simulink library "VehicleMdl"  (R2018b)
settings: Solver=VariableStepAuto  StartTime=0.0  StopTime=10.0  RelTol=1e-3
settings Model: Creator=Haraszti Sándor  LastModifiedBy=Haraszti Sándor

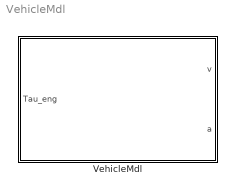
== system VehicleMdl ==
  VehicleMdl : Subsystem  mask{v_max=25, v_min=0, a_max=3, a_min=-3}
      mask prompts: v_max "v_max [m/s]"; v_min "v_min [m/s]"; a_max "a_max [m/s^2]"; a_min "a_min [m/s^2]"

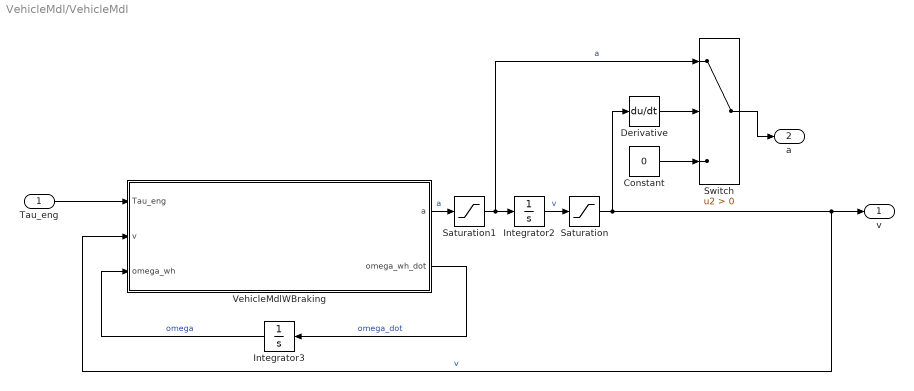
== system VehicleMdl/VehicleMdl ==
  Tau_eng : Inport
  Constant : Constant  Value=0
  Derivative : Derivative
  Integrator2 : Integrator
  Integrator3 : Integrator
  Saturation : Saturate  UpperLimit=v_max  LowerLimit=v_min
  Saturation1 : Saturate  UpperLimit=a_max  LowerLimit=a_min
  Switch : Switch  Criteria=u2 > Threshold
  VehicleMdlWBraking : MATLAB Function  TreatAsAtomicUnit=on
  v : Outport
  a : Outport  Port=2
  wires:
  Constant/1 -> Switch/3
  Switch/1 -> a/1
  Derivative/1 -> Switch/2
  Saturation1/1 -> Integrator2/1, Switch/1  "a"
  VehicleMdlWBraking/1(a) -> Saturation1/1  "a"
  VehicleMdlWBraking/2(omega_wh_dot) -> Integrator3/1  "omega_dot"
  Integrator3/1 -> VehicleMdlWBraking/3(omega_wh)  "omega"
  Saturation/1 -> Derivative/1, v/1, VehicleMdlWBraking/2(v)  "v"
  Tau_eng/1 -> VehicleMdlWBraking/1(Tau_eng)
  Integrator2/1 -> Saturation/1  "v"

== matlab function VehicleMdl/VehicleMdlWBraking ==
  data: Tau_eng input; a output; v input; omega_wh input; omega_wh_dot output
function [a, omega_wh_dot] = vehicleMdl(Tau_eng, v, omega_wh)
% The inputs of the system are:
%           the traction force
%           the braking force
% The measured signal:
%           longitudinal velocity of the vehicle.
% Prescribed Prformances:
%           The tracking of the reference longitudinal velocity
% Parameters:
%           A - front surface
%           m - total mass of the car
%           Cd - drag coefficient
%           Cr - rolling resistance coefficient
%           ri - effective wheel radius
%           Ji - wheel inertia
%           Cfi - rolling friction coefficient
%           rho - air density
%           v longitudinal velocity
    
    % Parameters - Opel Corsa 1.0i 12V (https://katalogus.hasznaltauto.hu/opel/opel_corsa_1.0i_12v_city-22413)
    m = 1320;                                   % [kg] full mass of the vehicle
    rho = 1.225;                                % [kg/m^3] air density
    A = 1.42*2.44;                              % [m^2]front surface of the vehicle
    C_d = 0.31;                                 % [-] drag coefficient (source: wikipedia https://en.wikipedia.org/wiki/Automobile_drag_coefficient )
    C_r = 0.015;                                % [-] rolling coefficient (source: wikipedia https://en.wikipedia.org/wiki/Rolling_resistance )
    r_wh = 21*10^(-2);                          % [m] radius of a wheel
    J = 1.5 * 10^(-3);                          % [kg * m^2] wheel inertia (??)
    C_f = C_r;                                  % [-] rolling friction coefficient
    
    % Calculate traction maximum torque on both rear wheel
    % braking flag: 1 if acceleration, -1 if brake
    brake_falg = sign(Tau_eng);
    Tau_tr = abs(Tau_eng*0.8);
    
    % Normal force of the vehicle
    F_z = m*9.81;
    % Calculationg adhesion coefficient with Magic-formula
    s = abs((v-omega_wh*r_wh)/(max(v, omega_wh*r_wh)));    %[-] wheel slip
    if isnan(s)
        s = 0;
    end
    % Magic-formula: D=1; C=3; B=5; E=1;
    mu = abs(sin(3*atan(5*s-(5*s-atan(5*s)))));
    
    % Decide wether it is slip or not
    % if slipping: F_tr > F_max
    if (Tau_tr/r_wh)>(mu*F_z)
        F_x = mu*F_z;
    else
        F_x = Tau_tr/r_wh;
    end
    
    % Resistance force calculation
    F_d = 0.5*rho*A*C_d*v^2;                    % [N] Drag resistance force
    R_xi = m*9.81*C_r;                          % [N] Rolling resistance force
    
    Tau_d = C_f * abs(omega_wh);
    
%     acceleration of the vehicle
%     if Tau_eng<0
%         F_x = mu*F_z;
%         Tau_tr = F_x*r_wh;
%     end
    a = brake_falg*abs((-F_x-F_d-R_xi)/m);
    
    % angular acceleration for velocity measurement
    omega_wh_dot = brake_falg*abs((Tau_eng+Tau_tr-Tau_d)/J);
end
